simulink model "geometria"  (R2022b)
settings: Solver=VariableStepAuto  StartTime=0.0  StopTime=10.0  RelTol=1e-3
values from neighbouring files (symbols this model uses):
  delta_h = (pi/2-alpha-acos((L^2+R^2-(Y+x+DeltaH).^2)/(2*L*R)))*180/pi    [funkcja_bloczka_geometria.m]
  x = -y_max/2:0.5:y_max/2    [funkcja_bloczka_geometria.m]
settings Model: Creator=Magda  LastModifiedBy=Magda

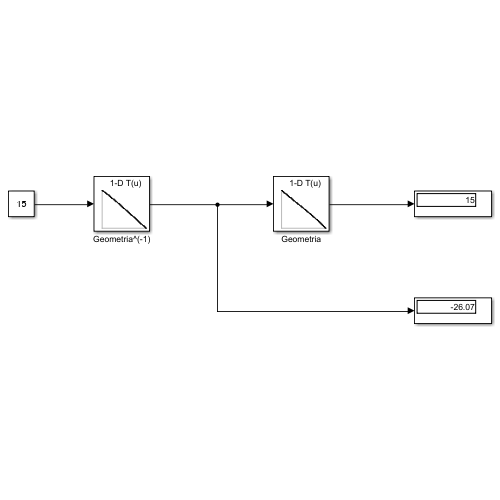
[thumbnail: Simulink's stored preview of the top-level diagram]
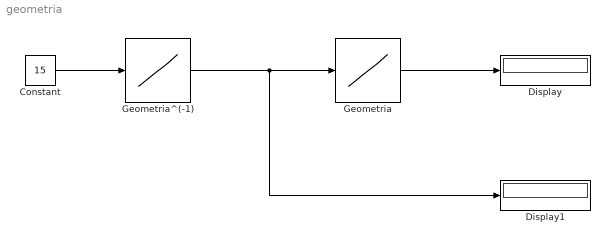
== system geometria ==
  Constant : Constant  Value=15
  Display : Display
  Display1 : Display
  Geometria : Lookup_n-D  NumberOfTableDimensions=1  BreakpointsForDimension1=x  Table=delta_h  InternalRulePriority=Speed  RndMeth=Simplest
  Geometria^(-1) : Lookup_n-D  NumberOfTableDimensions=1  BreakpointsForDimension1=flip(delta_h)  Table=flip(x)  InternalRulePriority=Speed  RndMeth=Simplest
  wires:
  Constant/1 -> Geometria^(-1)/1
  Geometria^(-1)/1 -> Display1/1, Geometria/1
  Geometria/1 -> Display/1
